simulink model "galton_mdl"  (Simulink 7.3)
settings: Solver=ode45  StartTime=0.0  StopTime=10.0  MaxStep=0.1  RelTol=1e-3
settings Model: Creator=zhan  LastModifiedBy=zhan
settings DataIOCC: FinalStateName=xF  SaveFinalState=on  SaveCompleteFinalSimState=on

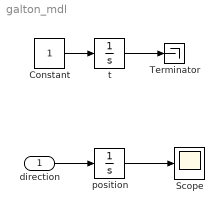
== system galton_mdl ==
  direction : Inport  OutDataType=fixdt(1, 16)  OutScaling=2^0  Interpolate=off
  Constant : Constant  OutDataType=fixdt(1, 16)  OutScaling=2^0
  Scope : Scope
      settings: YMin=0.095  YMax=0.105
  Terminator : Terminator
  position : Integrator
  t : Integrator
  wires:
  Constant/1 -> t/1
  t/1 -> Terminator/1
  direction/1 -> position/1
  position/1 -> Scope/1
